simulink model "bldc_sim_2024a_v3"  (R2024a)
settings: Solver=VariableStepAuto  StartTime=0.0  StopTime=0.5  FixedStep=1e-6  MaxStep=1e-4  RelTol=1e-3
values from neighbouring files (symbols this model uses):
  D_m = 1e-5    (= 1e-05)    [setup_motor_params.m]
  J = 12e-4    (= 0.0012)    [setup_motor_params.m]
  L_ss = 0.45e-3    (= 0.00045)    [setup_motor_params.m]
  lambda_m = 21.5e-3    (= 0.0215)    [setup_motor_params.m]
  P = 8    [setup_motor_params.m]
  phi_A_deg = 9.0 * 0    (= 0)    [setup_motor_params.m]
  phi_B_deg = -1.0 * 0    (= 0)    [setup_motor_params.m]
  phi_C_deg = 7.0* 0    (= 0)    [setup_motor_params.m]
  R_s = 0.15    [setup_motor_params.m]
  tau_s = L_ss/R_s    (= 0.003)    [setup_motor_params.m]
  Ts_motor = 1e-6    (= 1e-06)    [setup_motor_params.m]
undefined symbols (not defined in the file or in its folder): closed_loop, R_vs, V_bus
libraries: spsMosfetLib x6, spsSeriesRLCBranchLib x4, spsPWMGeneratorDCDCLib x3, spsVoltageMeasurementLib x3, spsControlledCurrentSourceLib x3, spsDCVoltageSourceLib x1, spspowerguiLib x1
settings Model: Creator=Aether  LastModifiedBy=Aether

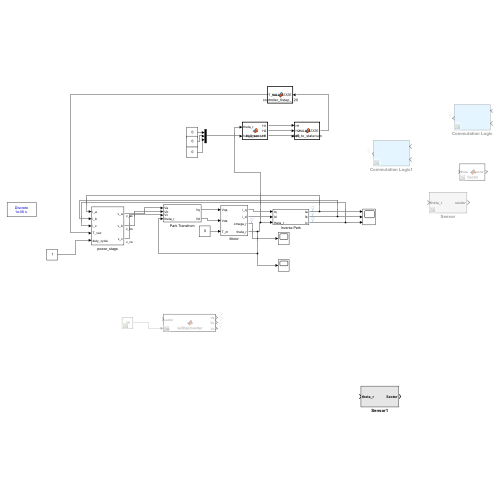
[thumbnail: Simulink's stored preview of the top-level diagram]
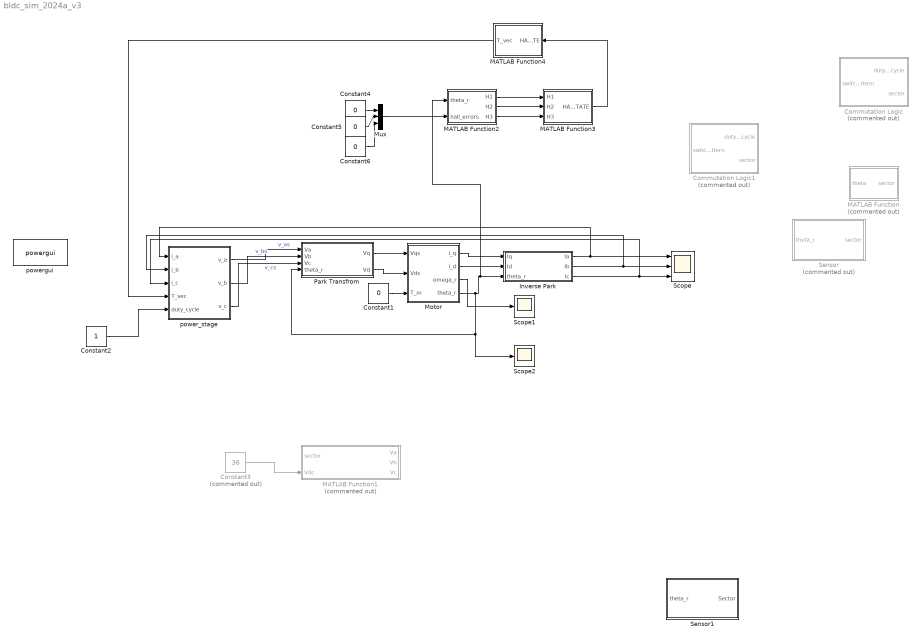
== system bldc_sim_2024a_v3 ==
  Commutation Logic : Subsystem  Commented=on
  Commutation Logic1 : Subsystem  Commented=on
  Constant{1,4..6} (4 alike) : Constant  Value=0
  Constant2 : Constant
  Constant3 : Constant  Commented=on  Value=36
  Inverse Park : Subsystem
  MATLAB Function : MATLAB Function  Commented=on  TreatAsAtomicUnit=on
  MATLAB Function1 : MATLAB Function  Commented=on  TreatAsAtomicUnit=on
  MATLAB Function2 : MATLAB Function  TreatAsAtomicUnit=on
  MATLAB Function3 : MATLAB Function  TreatAsAtomicUnit=on
  MATLAB Function4 : MATLAB Function  TreatAsAtomicUnit=on
  Motor : Subsystem
  Mux : Mux  Inputs=3
  Park Transfrom : Subsystem
  Scope : Scope  NumInputPorts=3
  Scope1 : Scope
  Scope2 : Scope
  Sensor : Subsystem  Commented=on
  Sensor1 : Subsystem
  power_stage : Subsystem
  powergui : spspowerguiLib/powergui  Priority=1  SimulationMode=Discrete  SampleTime=1e-6  frequency=60  Iterations=50  frequencyindice=0  Pbase=100e6  ErrMax=1e-4  UnitsV=kV  UnitsW=MW  buscounter=0  FunctionMessages=off  echomessages=off  EnableUseOfTLC=off  CurrentSourceSwitches=off  DisableSnubberDevices=off  DisableRonSwitches=off  DisableVfSwitches=off  DisplayEquations=off  AutomaticDiscreteSolvers=off  SolverType=Tustin/Backward Euler (TBE)  Interpol=off  ExternalGateDelay=off  methode=off  Ts=100  x0status=blocks  SPID=on  SwTol=0  HookPort=off  NonlinearTolerance=1e-4  nMaxIteration=100  ContinueOnMaxIteration=off  RestoreLinks=warning  ResistiveCurrentMeasurement=off  Frange=[0:2:500]  Ylog=off  Xlog=on  ShowGrid=off  save=off  variable=ZData  structure=0  ZoomFFT=off  StartTime=0.0  cycles=1  DisplayStyle=1  fundamental=60  FreqAxis=off  MaxFrequency=1000  frequencyindicesteady=1  RmsSteady=1  display=off
  wires:
  Park Transfrom/1(Vq) -> Motor/1(Vqs)
  Park Transfrom/2(Vd) -> Motor/2(Vds)
  Motor/1(i_q) -> Inverse Park/1(Iq)
  Motor/2(i_d) -> Inverse Park/2(Id)
  Motor/4(theta_r) -> Scope2/1, Park Transfrom/4(theta_r), MATLAB Function2/1(theta_r), Inverse Park/3(theta_r)
  Inverse Park/1(Ia) -> power_stage/1(i_a), Scope/1
  Inverse Park/2(Ib) -> power_stage/2(i_b), Scope/2
  Inverse Park/3(Ic) -> power_stage/3(i_c), Scope/3
  Constant1/1 -> Motor/3(T_m)
  Motor/3(omega_r) -> Scope1/1
  Constant3/1 -> MATLAB Function1/2(Vdc)
  MATLAB Function4/1(T_vec) -> power_stage/4(T_vec)
  Constant6/1 -> Mux/3
  Constant4/1 -> Mux/1
  MATLAB Function2/1(H1) -> MATLAB Function3/1(H1)
  Mux/1 -> MATLAB Function2/2(hall_errors)
  MATLAB Function2/3(H3) -> MATLAB Function3/3(H3)
  MATLAB Function3/1(HALL_STATE) -> MATLAB Function4/1(HALL_STATE)
  Constant5/1 -> Mux/2
  MATLAB Function2/2(H2) -> MATLAB Function3/2(H2)
  power_stage/1(v_a) -> Park Transfrom/1(Va)  "v_as"
  power_stage/2(v_b) -> Park Transfrom/2(Vb)  "v_bs"
  power_stage/3(v_c) -> Park Transfrom/3(Vc)  "v_cs"
  Constant2/1 -> power_stage/5(duty_cycle)

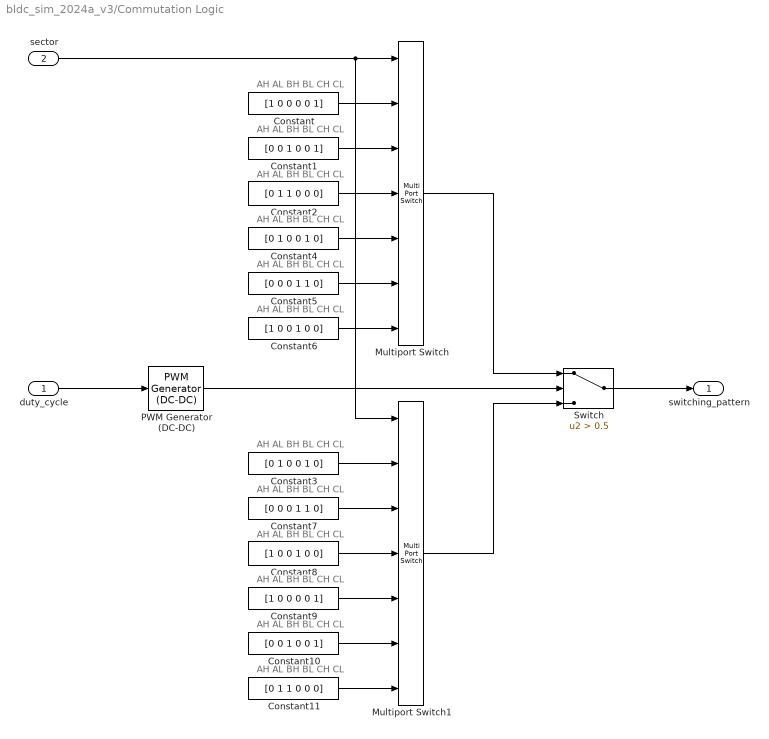
== system bldc_sim_2024a_v3/Commutation Logic ==
  note: AH AL BH BL CH CL
  note: AH AL BH BL CH CL
  note: AH AL BH BL CH CL
  note: AH AL BH BL CH CL
  note: AH AL BH BL CH CL
  note: AH AL BH BL CH CL
  note: AH AL BH BL CH CL
  note: AH AL BH BL CH CL
  note: AH AL BH BL CH CL
  note: AH AL BH BL CH CL
  note: AH AL BH BL CH CL
  note: AH AL BH BL CH CL
  duty_cycle : Inport
  sector : Inport  Port=2
  Constant : Constant  Value=[1 0 0 0 0 1]
  Constant1 : Constant  Value=[0 0 1 0 0 1]
  Constant10 : Constant  Value=[0 0 1 0 0 1]
  Constant11 : Constant  Value=[0 1 1 0 0 0]
  Constant2 : Constant  Value=[0 1 1 0 0 0]
  Constant3 : Constant  Value=[0 1 0 0 1 0]
  Constant4 : Constant  Value=[0 1 0 0 1 0]
  Constant5 : Constant  Value=[0 0 0 1 1 0]
  Constant6 : Constant  Value=[1 0 0 1 0 0]
  Constant7 : Constant  Value=[0 0 0 1 1 0]
  Constant8 : Constant  Value=[1 0 0 1 0 0]
  Constant9 : Constant  Value=[1 0 0 0 0 1]
  Multiport Switch : MultiPortSwitch  Inputs=6  SaturateOnIntegerOverflow=off  InputSameDT=off
  Multiport Switch1 : MultiPortSwitch  Inputs=6  SaturateOnIntegerOverflow=off  InputSameDT=off
  PWM Generator (DC-DC) : spsPWMGeneratorDCDCLib/PWM Generator (DC-DC)  Fsw=1e4  Ts=Ts_motor
  Switch : Switch  Criteria=u2 > Threshold  Threshold=0.5  SaturateOnIntegerOverflow=off  InputSameDT=off
  "  switching_pattern" : Outport  VectorParamsAs1DForOutWhenUnconnected=off
  wires:
  Constant6/1 -> Multiport Switch/7
  Constant4/1 -> Multiport Switch/5
  sector/1 -> Multiport Switch1/1, Multiport Switch/1
  Constant1/1 -> Multiport Switch/3
  Constant2/1 -> Multiport Switch/4
  Constant5/1 -> Multiport Switch/6
  Constant/1 -> Multiport Switch/2
  Constant9/1 -> Multiport Switch1/5
  Constant11/1 -> Multiport Switch1/7
  Constant3/1 -> Multiport Switch1/2
  Constant7/1 -> Multiport Switch1/3
  Constant10/1 -> Multiport Switch1/6
  Constant8/1 -> Multiport Switch1/4
  PWM Generator (DC-DC)/1 -> Switch/2
  Switch/1 -> "  switching_pattern"/1
  Multiport Switch/1 -> Switch/1
  Multiport Switch1/1 -> Switch/3
  duty_cycle/1 -> PWM Generator (DC-DC)/1

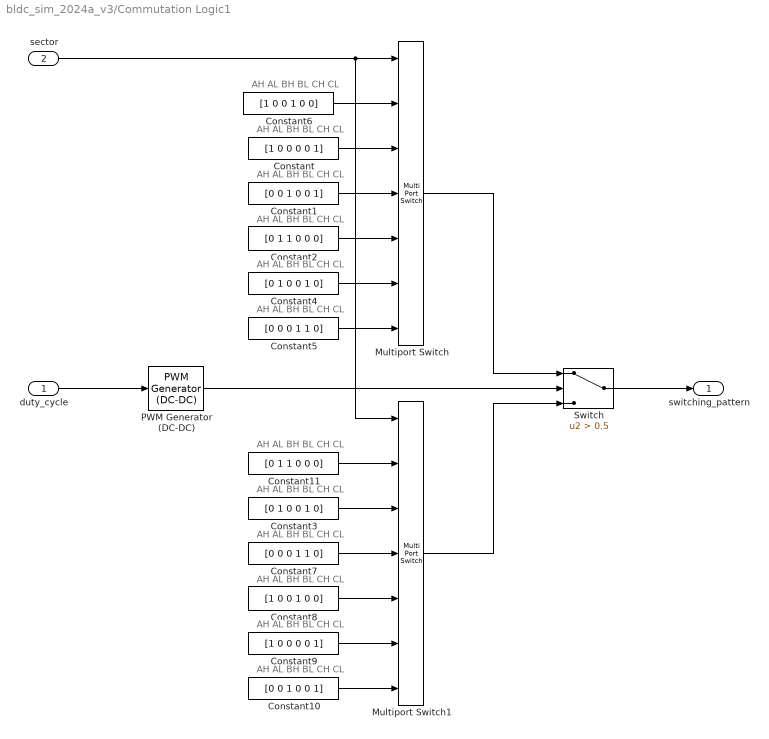
== system bldc_sim_2024a_v3/Commutation Logic1 ==
  note: AH AL BH BL CH CL
  note: AH AL BH BL CH CL
  note: AH AL BH BL CH CL
  note: AH AL BH BL CH CL
  note: AH AL BH BL CH CL
  note: AH AL BH BL CH CL
  note: AH AL BH BL CH CL
  note: AH AL BH BL CH CL
  note: AH AL BH BL CH CL
  note: AH AL BH BL CH CL
  note: AH AL BH BL CH CL
  note: AH AL BH BL CH CL
  duty_cycle : Inport
  sector : Inport  Port=2
  Constant : Constant  Value=[1 0 0 0 0 1]
  Constant1 : Constant  Value=[0 0 1 0 0 1]
  Constant10 : Constant  Value=[0 0 1 0 0 1]
  Constant11 : Constant  Value=[0 1 1 0 0 0]
  Constant2 : Constant  Value=[0 1 1 0 0 0]
  Constant3 : Constant  Value=[0 1 0 0 1 0]
  Constant4 : Constant  Value=[0 1 0 0 1 0]
  Constant5 : Constant  Value=[0 0 0 1 1 0]
  Constant6 : Constant  Value=[1 0 0 1 0 0]
  Constant7 : Constant  Value=[0 0 0 1 1 0]
  Constant8 : Constant  Value=[1 0 0 1 0 0]
  Constant9 : Constant  Value=[1 0 0 0 0 1]
  Multiport Switch : MultiPortSwitch  Inputs=6  SaturateOnIntegerOverflow=off  InputSameDT=off
  Multiport Switch1 : MultiPortSwitch  Inputs=6  SaturateOnIntegerOverflow=off  InputSameDT=off
  PWM Generator (DC-DC) : spsPWMGeneratorDCDCLib/PWM Generator (DC-DC)  Fsw=1e4  Ts=Ts_motor
  Switch : Switch  Criteria=u2 > Threshold  Threshold=0.5  SaturateOnIntegerOverflow=off  InputSameDT=off
  "  switching_pattern" : Outport  VectorParamsAs1DForOutWhenUnconnected=off
  wires:
  sector/1 -> Multiport Switch1/1, Multiport Switch/1
  PWM Generator (DC-DC)/1 -> Switch/2
  Switch/1 -> "  switching_pattern"/1
  Multiport Switch/1 -> Switch/1
  Multiport Switch1/1 -> Switch/3
  duty_cycle/1 -> PWM Generator (DC-DC)/1
  Constant5/1 -> Multiport Switch/7
  Constant4/1 -> Multiport Switch/6
  Constant2/1 -> Multiport Switch/5
  Constant1/1 -> Multiport Switch/4
  Constant/1 -> Multiport Switch/3
  Constant6/1 -> Multiport Switch/2
  Constant10/1 -> Multiport Switch1/7
  Constant9/1 -> Multiport Switch1/6
  Constant8/1 -> Multiport Switch1/5
  Constant7/1 -> Multiport Switch1/4
  Constant3/1 -> Multiport Switch1/3
  Constant11/1 -> Multiport Switch1/2

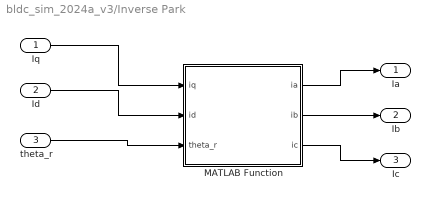
== system bldc_sim_2024a_v3/Inverse Park ==
  Iq : Inport
  Id : Inport  Port=2
  theta_r : Inport  Port=3
  MATLAB Function : MATLAB Function  TreatAsAtomicUnit=on
  Ia : Outport
  Ib : Outport  Port=2
  Ic : Outport  Port=3
  wires:
  theta_r/1 -> MATLAB Function/3(theta_r)
  Id/1 -> MATLAB Function/2(id)
  Iq/1 -> MATLAB Function/1(iq)
  MATLAB Function/3(ic) -> Ic/1
  MATLAB Function/1(ia) -> Ia/1
  MATLAB Function/2(ib) -> Ib/1

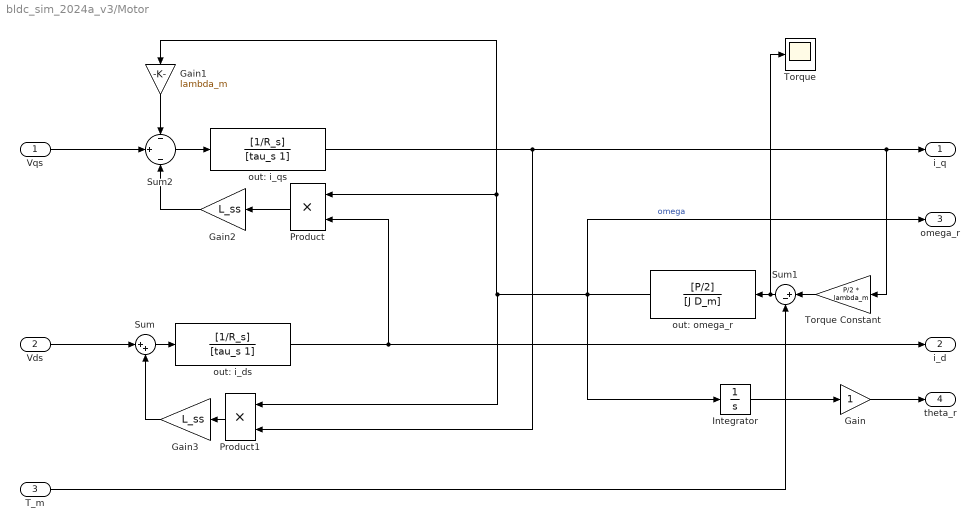
== system bldc_sim_2024a_v3/Motor ==
  Vqs : Inport
  Vds : Inport  Port=2
  T_m : Inport  Port=3
  Gain : Gain
  Gain1 : Gain  Gain=lambda_m
  Gain2 : Gain  Gain=L_ss
  Gain3 : Gain  Gain=L_ss
  Integrator : Integrator
  Product : Product
  Product1 : Product
  Sum : Sum  Inputs=|++
  Sum1 : Sum  Inputs=|+-
  Sum2 : Sum  Inputs=-|+|-
  Torque : Scope
  Torque Constant : Gain  Gain=P/2 * lambda_m
  out: i_ds : TransferFcn  Numerator=[1/R_s]  Denominator=[tau_s 1]
  out: i_qs : TransferFcn  Numerator=[1/R_s]  Denominator=[tau_s 1]
  out: omega_r : TransferFcn  Numerator=[P/2]  Denominator=[J D_m]
  i_q : Outport
  i_d : Outport  Port=2
  omega_r : Outport  Port=3
  theta_r : Outport  Port=4
  wires:
  Sum2/1 -> out: i_qs/1
  Vqs/1 -> Sum2/2
  out: omega_r/1 -> omega_r/1, Integrator/1, Product1/1, Product/1, Gain1/1  "omega"
  Gain1/1 -> Sum2/1
  out: i_ds/1 -> Product/2, i_d/1
  Integrator/1 -> Gain/1
  T_m/1 -> Sum1/2
  Sum1/1 -> Torque/1, out: omega_r/1
  Sum/1 -> out: i_ds/1
  Torque Constant/1 -> Sum1/1
  Product/1 -> Gain2/1
  out: i_qs/1 -> Product1/2, i_q/1, Torque Constant/1
  Vds/1 -> Sum/1
  Gain/1 -> theta_r/1
  Product1/1 -> Gain3/1
  Gain3/1 -> Sum/2
  Gain2/1 -> Sum2/3

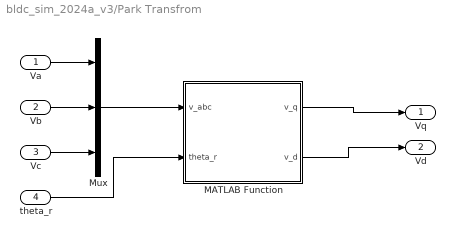
== system bldc_sim_2024a_v3/Park Transfrom ==
  Va : Inport
  Vb : Inport  Port=2
  Vc : Inport  Port=3
  theta_r : Inport  Port=4
  MATLAB Function : MATLAB Function  TreatAsAtomicUnit=on
  Mux : Mux  Inputs=3
  Vq : Outport
  Vd : Outport  Port=2
  wires:
  theta_r/1 -> MATLAB Function/2(theta_r)
  Vb/1 -> Mux/2
  Va/1 -> Mux/1
  Vc/1 -> Mux/3
  Mux/1 -> MATLAB Function/1(v_abc)
  MATLAB Function/2(v_d) -> Vd/1
  MATLAB Function/1(v_q) -> Vq/1

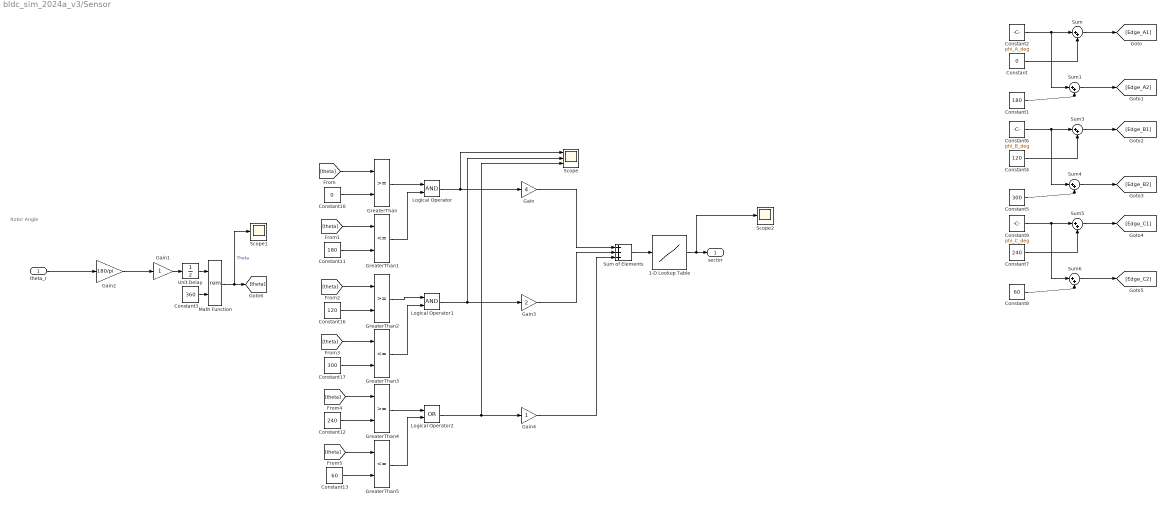
== system bldc_sim_2024a_v3/Sensor ==
  note: Rotor Angle
  theta_r : Inport
  1-D Lookup Table : Lookup_n-D  NumberOfTableDimensions=1  BreakpointsForDimension1=[1 2 3 4 5 6]  Table=[6 4 5 2 1 3]  ExtrapMethod=Clip  InternalRulePriority=Speed  RndMeth=Simplest
  Constant : Constant  Value=0
  Constant1 : Constant  Value=180
  Constant10 : Constant  Value=0
  Constant11 : Constant  Value=180
  Constant12 : Constant  Value=240
  Constant13 : Constant  Value=60
  Constant16 : Constant  Value=120
  Constant17 : Constant  Value=300
  Constant2 : Constant  Value=phi_A_deg
  Constant3 : Constant  Value=360
  Constant4 : Constant  Value=120
  Constant5 : Constant  Value=300
  Constant6 : Constant  Value=phi_B_deg
  Constant7 : Constant  Value=240
  Constant8 : Constant  Value=60
  Constant9 : Constant  Value=phi_C_deg
  Gain : Gain  Gain=4
  Gain1 : Gain
  Gain2 : Gain  Gain=180/pi
  Gain3 : Gain  Gain=2
  Gain4 : Gain
  GreaterThan : RelationalOperator  OutDataTypeStr=boolean  RndMeth=Simplest  InputSameDT=off
  GreaterThan1 : RelationalOperator  Operator=<=  OutDataTypeStr=boolean  RndMeth=Simplest  InputSameDT=off
  GreaterThan2 : RelationalOperator  OutDataTypeStr=boolean  RndMeth=Simplest  InputSameDT=off
  GreaterThan3 : RelationalOperator  Operator=<=  OutDataTypeStr=boolean  RndMeth=Simplest  InputSameDT=off
  GreaterThan4 : RelationalOperator  OutDataTypeStr=boolean  RndMeth=Simplest  InputSameDT=off
  GreaterThan5 : RelationalOperator  Operator=<=  OutDataTypeStr=boolean  RndMeth=Simplest  InputSameDT=off
  Logical Operator : Logic  AllPortsSameDT=off  OutDataTypeStr=boolean
  Logical Operator1 : Logic  AllPortsSameDT=off  OutDataTypeStr=boolean
  Logical Operator2 : Logic  Operator=OR  AllPortsSameDT=off  OutDataTypeStr=boolean
  Math Function : Math  Operator=rem  SignedPower=on
  Scope : Scope  NumInputPorts=3
  Scope1 : Scope
  Scope2 : Scope
  Sum{,1,3..6} (6 alike) : Sum  Inputs=|++
  Sum of Elements : Sum  Inputs=+++
  Unit Delay : UnitDelay  SampleTime=Ts_motor  HasFrameUpgradeWarning=on
  sector : Outport
  wires:
  Gain2/1 -> Gain1/1
  Constant3/1 -> Math Function/2
  Gain1/1 -> Unit Delay/1
  Unit Delay/1 -> Math Function/1
  Constant/1 -> Sum/2
  Constant2/1 -> Sum1/1, Sum/1
  Constant1/1 -> Sum1/2
  Sum/1 -> [Edge_A1]
  Sum1/1 -> [Edge_A2]
  Constant6/1 -> Sum4/1, Sum3/1
  Constant5/1 -> Sum4/2
  Constant4/1 -> Sum3/2
  Sum3/1 -> [Edge_B1]
  Sum4/1 -> [Edge_B2]
  Constant9/1 -> Sum6/1, Sum5/1
  Constant8/1 -> Sum6/2
  Constant7/1 -> Sum5/2
  Sum5/1 -> [Edge_C1]
  Sum6/1 -> [Edge_C2]
  theta_r/1 -> Gain2/1
  Math Function/1 -> Scope1/1, [theta]  "Theta"
  GreaterThan/1 -> Logical Operator/1
  [theta] -> GreaterThan/1
  Constant11/1 -> GreaterThan1/2
  GreaterThan1/1 -> Logical Operator/2
  GreaterThan3/1 -> Logical Operator1/2
  GreaterThan2/1 -> Logical Operator1/1
  GreaterThan4/1 -> Logical Operator2/1
  GreaterThan5/1 -> Logical Operator2/2
  Logical Operator/1 -> Scope/1, Gain/1
  Logical Operator1/1 -> Scope/2, Gain3/1
  Logical Operator2/1 -> Scope/3, Gain4/1
  Sum of Elements/1 -> 1-D Lookup Table/1
  Gain/1 -> Sum of Elements/1
  Gain3/1 -> Sum of Elements/2
  Gain4/1 -> Sum of Elements/3
  1-D Lookup Table/1 -> Scope2/1, sector/1
  Constant10/1 -> GreaterThan/2
  [theta] -> GreaterThan1/1
  [theta] -> GreaterThan2/1
  Constant16/1 -> GreaterThan2/2
  [theta] -> GreaterThan3/1
  Constant17/1 -> GreaterThan3/2
  [theta] -> GreaterThan4/1
  Constant12/1 -> GreaterThan4/2
  [theta] -> GreaterThan5/1
  Constant13/1 -> GreaterThan5/2

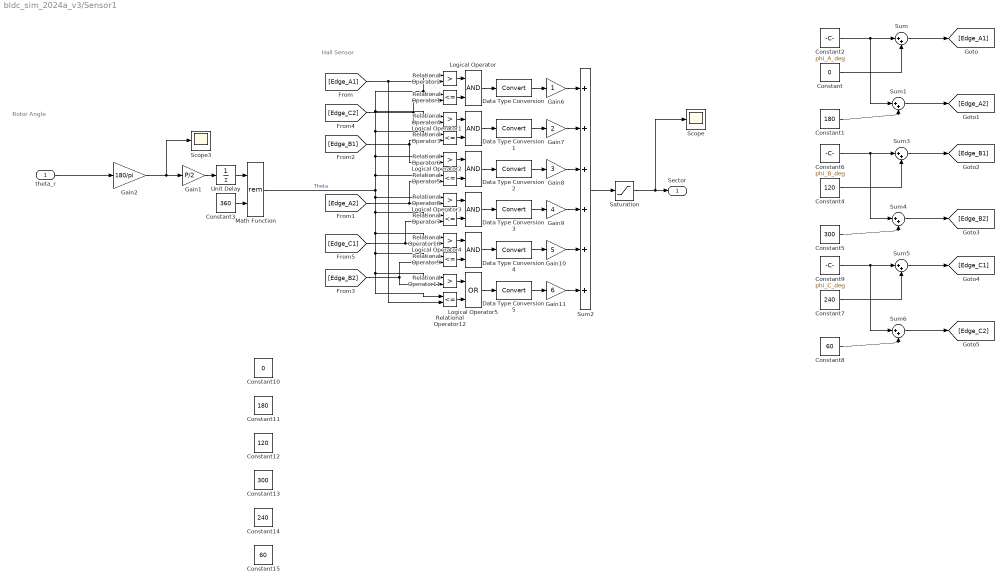
== system bldc_sim_2024a_v3/Sensor1 ==
  note: Rotor Angle
  note: Hall Sensor
  theta_r : Inport
  Constant : Constant  Value=0
  Constant1 : Constant  Value=180
  Constant10 : Constant  Value=0
  Constant11 : Constant  Value=180
  Constant12 : Constant  Value=120
  Constant13 : Constant  Value=300
  Constant14 : Constant  Value=240
  Constant15 : Constant  Value=60
  Constant2 : Constant  Value=phi_A_deg
  Constant3 : Constant  Value=360
  Constant4 : Constant  Value=120
  Constant5 : Constant  Value=300
  Constant6 : Constant  Value=phi_B_deg
  Constant7 : Constant  Value=240
  Constant8 : Constant  Value=60
  Constant9 : Constant  Value=phi_C_deg
  Data Type Conversion{,1..5} (6 alike) : DataTypeConversion
  Gain1 : Gain  Gain=P/2
  Gain10 : Gain  Gain=5  SaturateOnIntegerOverflow=on  OutDataTypeStr=Inherit: Same as input  ParamDataTypeStr=Inherit: Same as input
  Gain11 : Gain  Gain=6  SaturateOnIntegerOverflow=on  OutDataTypeStr=Inherit: Same as input  ParamDataTypeStr=Inherit: Same as input
  Gain2 : Gain  Gain=180/pi
  Gain6 : Gain  SaturateOnIntegerOverflow=on  OutDataTypeStr=Inherit: Same as input  ParamDataTypeStr=Inherit: Same as input
  Gain7 : Gain  Gain=2  SaturateOnIntegerOverflow=on  OutDataTypeStr=Inherit: Same as input  ParamDataTypeStr=Inherit: Same as input
  Gain8 : Gain  Gain=3  SaturateOnIntegerOverflow=on  OutDataTypeStr=Inherit: Same as input  ParamDataTypeStr=Inherit: Same as input
  Gain9 : Gain  Gain=4  SaturateOnIntegerOverflow=on  OutDataTypeStr=Inherit: Same as input  ParamDataTypeStr=Inherit: Same as input
  Logical Operator{,1..4} (5 alike) : Logic
  Logical Operator5 : Logic  Operator=OR
  Math Function : Math  Operator=rem  SignedPower=on
  Relational Operator{1,3,5,7,9,12} (6 alike) : RelationalOperator  Operator=<=
  Relational Operator{2,4,6,8,10..11} (6 alike) : RelationalOperator  Operator=>
  Saturation : Saturate  UpperLimit=6  LowerLimit=1
  Scope : Scope
  Scope3 : Scope
  Sum{,1,3..6} (6 alike) : Sum  Inputs=|++
  Sum2 : Sum  Inputs=++++++  InputSameDT=on  SaturateOnIntegerOverflow=on  OutDataTypeStr=Inherit: Same as first input
  Unit Delay : UnitDelay  SampleTime=Ts_motor  HasFrameUpgradeWarning=on
  Sector : Outport
  wires:
  Saturation/1 -> Scope/1, Sector/1
  Math Function/1 -> Relational Operator2/1, Relational Operator1/1, Relational Operator4/1, Relational Operator3/1, Relational Operator6/1, Relational Operator5/1, Relational Operator12/1, Relational Operator11/1, Relational Operator9/1, Relational Operator10/1, Relational Operator7/1, Relational Operator8/1  "Theta"
  Data Type Conversion5/1 -> Gain11/1
  Data Type Conversion4/1 -> Gain10/1
  Data Type Conversion3/1 -> Gain9/1
  Data Type Conversion2/1 -> Gain8/1
  Data Type Conversion1/1 -> Gain7/1
  Data Type Conversion/1 -> Gain6/1
  Relational Operator2/1 -> Logical Operator/1
  Relational Operator1/1 -> Logical Operator/2
  Logical Operator/1 -> Data Type Conversion/1
  [Edge_A1] -> Relational Operator12/2, Relational Operator2/2
  Relational Operator4/1 -> Logical Operator1/1
  Relational Operator3/1 -> Logical Operator1/2
  Logical Operator1/1 -> Data Type Conversion1/1
  [Edge_C2] -> Relational Operator1/2, Relational Operator4/2
  Relational Operator6/1 -> Logical Operator2/1
  Relational Operator5/1 -> Logical Operator2/2
  Logical Operator2/1 -> Data Type Conversion2/1
  Relational Operator8/1 -> Logical Operator3/1
  Relational Operator7/1 -> Logical Operator3/2
  Logical Operator3/1 -> Data Type Conversion3/1
  Relational Operator10/1 -> Logical Operator4/1
  Relational Operator9/1 -> Logical Operator4/2
  Logical Operator4/1 -> Data Type Conversion4/1
  Relational Operator11/1 -> Logical Operator5/1
  Relational Operator12/1 -> Logical Operator5/2
  Logical Operator5/1 -> Data Type Conversion5/1
  Gain6/1 -> Sum2/1
  Gain7/1 -> Sum2/2
  Gain8/1 -> Sum2/3
  Gain9/1 -> Sum2/4
  Gain10/1 -> Sum2/5
  Gain11/1 -> Sum2/6
  Sum2/1 -> Saturation/1
  Gain2/1 -> Scope3/1, Gain1/1
  Constant3/1 -> Math Function/2
  Gain1/1 -> Unit Delay/1
  Unit Delay/1 -> Math Function/1
  Constant/1 -> Sum/2
  Constant2/1 -> Sum1/1, Sum/1
  Constant1/1 -> Sum1/2
  Sum/1 -> [Edge_A1]
  Sum1/1 -> [Edge_A2]
  Constant6/1 -> Sum4/1, Sum3/1
  Constant5/1 -> Sum4/2
  Constant4/1 -> Sum3/2
  Sum3/1 -> [Edge_B1]
  Sum4/1 -> [Edge_B2]
  Constant9/1 -> Sum6/1, Sum5/1
  Constant8/1 -> Sum6/2
  Constant7/1 -> Sum5/2
  Sum5/1 -> [Edge_C1]
  Sum6/1 -> [Edge_C2]
  [Edge_B1] -> Relational Operator3/2, Relational Operator6/2
  [Edge_A2] -> Relational Operator5/2, Relational Operator8/2
  [Edge_C1] -> Relational Operator7/2, Relational Operator10/2
  [Edge_B2] -> Relational Operator11/2, Relational Operator9/2
  theta_r/1 -> Gain2/1

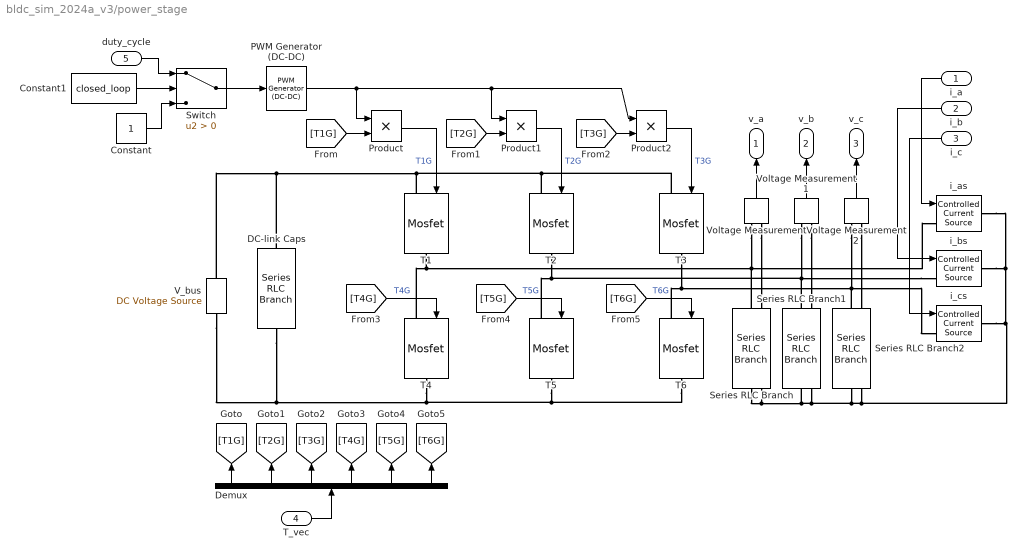
== system bldc_sim_2024a_v3/power_stage ==
  i_a : Inport
  i_b : Inport  Port=2
  i_c : Inport  Port=3
  T_vec : Inport  Port=4
  duty_cycle : Inport  Port=5
  Constant : Constant
  Constant1 : Constant  Value=closed_loop
  DC-link Caps : spsSeriesRLCBranchLib/Series RLC Branch  LConnTagsString=__new0  RConnTagsString=__new0  BranchType=RC  Resistance=1e-6  Inductance=0  SetiL0=off  InitialCurrent=0  Capacitance=100e-6  Setx0=off  InitialVoltage=0  Measurements=None
  Demux : Demux  Outputs=6
  PWM Generator (DC-DC) : spsPWMGeneratorDCDCLib/PWM Generator (DC-DC)  Fsw=f_SW_Hz  Ts=0
  Product : Product
  Product1 : Product
  Product2 : Product
  Series RLC Branch : spsSeriesRLCBranchLib/Series RLC Branch  LConnTagsString=__new0  RConnTagsString=__new0  BranchType=R  Resistance=R_vs  Inductance=0  SetiL0=off  InitialCurrent=0  Capacitance=inf  Setx0=off  InitialVoltage=0  Measurements=None
  Series RLC Branch1 : spsSeriesRLCBranchLib/Series RLC Branch  LConnTagsString=__new0  RConnTagsString=__new0  BranchType=R  Resistance=R_vs  Inductance=0  SetiL0=off  InitialCurrent=0  Capacitance=inf  Setx0=off  InitialVoltage=0  Measurements=None
  Series RLC Branch2 : spsSeriesRLCBranchLib/Series RLC Branch  LConnTagsString=__new0  RConnTagsString=__new0  BranchType=R  Resistance=R_vs  Inductance=0  SetiL0=off  InitialCurrent=0  Capacitance=inf  Setx0=off  InitialVoltage=0  Measurements=None
  Switch : Switch  Criteria=u2 > Threshold  SaturateOnIntegerOverflow=off  InputSameDT=off
  T{1..6} (6 alike) : spsMosfetLib/Mosfet  Ron=R_dsON_Ohm  Lon=0  Rd=0.01  Vfd=0.7  IC=0  Rs=1e5  Cs=inf  Measurements=off
  V_bus : spsDCVoltageSourceLib/DC Voltage Source  Amplitude=V_bus  Measurements=None
  Voltage Measurement : spsVoltageMeasurementLib/Voltage Measurement  PhasorSimulation=off  OutputType=Complex  PSBequivalent=0
  Voltage Measurement1 : spsVoltageMeasurementLib/Voltage Measurement  PhasorSimulation=off  OutputType=Complex  PSBequivalent=0
  Voltage Measurement2 : spsVoltageMeasurementLib/Voltage Measurement  PhasorSimulation=off  OutputType=Complex  PSBequivalent=0
  i_as : spsControlledCurrentSourceLib/Controlled Current Source  Initialize=on  Source_Type=AC  Amplitude=0  Phase=0  Frequency=0  Measurements=None
  i_bs : spsControlledCurrentSourceLib/Controlled Current Source  Initialize=on  Source_Type=AC  Amplitude=0  Phase=0  Frequency=0  Measurements=None
  i_cs : spsControlledCurrentSourceLib/Controlled Current Source  Initialize=on  Source_Type=AC  Amplitude=0  Phase=0  Frequency=0  Measurements=None
  v_a : Outport
  v_b : Outport  Port=2
  v_c : Outport  Port=3
  wires:
  T_vec/1 -> Demux/1
  Product1/1 -> T2/1  "T2G"
  PWM Generator (DC-DC)/1 -> Product/1, Product2/1, Product1/1
  Demux/6 -> [T6G]
  [T4G] -> T4/1  "T4G"
  [T5G] -> T5/1  "T5G"
  Demux/4 -> [T4G]
  Voltage Measurement/1 -> v_a/1
  [T2G] -> Product1/2
  Voltage Measurement1/1 -> v_b/1
  Voltage Measurement2/1 -> v_c/1
  i_a/1 -> i_as/1
  Demux/1 -> [T1G]
  Demux/5 -> [T5G]
  [T6G] -> T6/1  "T6G"
  i_c/1 -> i_cs/1
  Product/1 -> T1/1  "T1G"
  [T3G] -> Product2/2
  i_b/1 -> i_bs/1
  Product2/1 -> T3/1  "T3G"
  Demux/2 -> [T2G]
  Demux/3 -> [T3G]
  [T1G] -> Product/2
  duty_cycle/1 -> Switch/1
  Constant/1 -> Switch/3
  Constant1/1 -> Switch/2
  Switch/1 -> PWM Generator (DC-DC)/1
  connections:
  i_bs/LConn1 -- Voltage Measurement1/LConn1 -- Series RLC Branch1/LConn1 -- T2/RConn1 -- T5/LConn1
  DC-link Caps/RConn1 -- V_bus/LConn1 -- T4/RConn1 -- T6/RConn1 -- T5/RConn1
  DC-link Caps/LConn1 -- V_bus/RConn1 -- T1/LConn1 -- T3/LConn1 -- T2/LConn1
  T4/LConn1 -- T1/RConn1 -- Voltage Measurement/LConn1 -- Series RLC Branch/LConn1 -- i_as/LConn1
  T3/RConn1 -- T6/LConn1 -- Voltage Measurement2/LConn1 -- Series RLC Branch2/LConn1 -- i_cs/LConn1
  Series RLC Branch/RConn1 -- Voltage Measurement/LConn2 -- i_bs/RConn1 -- i_as/RConn1 -- i_cs/RConn1 -- Voltage Measurement2/LConn2 -- Series RLC Branch2/RConn1 -- Voltage Measurement1/LConn2 -- Series RLC Branch1/RConn1

== matlab function bldc_sim_2024a_v3/Inverse Park/MATLAB Function ==
  data: iq input; id input; ia output; theta_r input; ib output; ic output
function [ia, ib, ic] = inverse_park_transform(iq, id,theta_r)


th = theta_r;

K_inv = [ cos(th)                  sin(th);
          cos(th - 2*pi/3)         sin(th - 2*pi/3);
          cos(th + 2*pi/3)         sin(th + 2*pi/3) ];

i_dq = [iq; id];
i_abc = K_inv * i_dq;
ia = i_abc(1);
ib = i_abc(2);
ic = i_abc(3);

% a = 2*pi/3;
% K_inv = [cos(theta), sin(theta);
%          cos(theta-a), sin(theta-a);
%          cos(theta+a), sin(theta+a)];
% fqd_vec = [fq; fd];
% fs_vec = K_inv*fqd_vec;
% fa = fs_vec(1);
% fb = fs_vec(2);
% fc = fs_vec(3);


end

== matlab function bldc_sim_2024a_v3/Park Transfrom/MATLAB Function ==
  data: v_abc input; v_q output; theta_r input; v_d output
function [v_q, v_d] = park_transform(v_abc,theta_r)

th = theta_r;

K = (2/3) * [ cos(th)     cos(th - 2*pi/3)     cos(th + 2*pi/3); 
              sin(th)    sin(th - 2*pi/3)    sin(th + 2*pi/3) ];

v_dq = K * v_abc;

v_q = v_dq(1);
v_d = v_dq(2);
% %   Detailed explanation goes here
% a = 2*pi/3;
% K = (2/3)*[cos(theta), cos(theta-a), cos(theta+a);
%            sin(theta), sin(theta-a), sin(theta+a)];
% fs_vec = [fa, fb, fc]';
% fqd_vec = K*fs_vec;
% fq = fqd_vec(1);
% fd = fqd_vec(2);

end

== matlab function bldc_sim_2024a_v3/MATLAB Function ==
  data: theta input; sector output
function sector = Sector(theta)

P = 8;
theta = mod(theta * P/2, 2*pi); % wrap around

if theta >= 0 && theta < pi/3
    sector = 1;
elseif theta >= pi/3 && theta < 2*pi/3
    sector = 2;
elseif theta >= 2*pi/3 && theta < pi
    sector = 3;
elseif theta >= pi && theta < 4*pi/3
    sector = 4;
elseif theta >= 4*pi/3 && theta < 5*pi/3
    sector = 5;
else
    sector = 6;
end

== matlab function bldc_sim_2024a_v3/MATLAB Function1 ==
  data: sector input; Va output; Vdc input; Vb output; Vc output
function [Va, Vb, Vc] = sixStepInverter(sector, Vdc)

    states = int8([ 1 -1  0;   % sector 1
                    1  0 -1;   % sector 2
                    0  1 -1;   % sector 3
                   -1  1  0;   % sector 4
                   -1  0  1;   % sector 5
                    0 -1  1]); % sector 6


    

    Va = double(states(sector,1)) * (Vdc/2);
    Vb = double(states(sector,2)) * (Vdc/2);
    Vc = double(states(sector,3)) * (Vdc/2);
end

== matlab function bldc_sim_2024a_v3/MATLAB Function2 ==
  data: theta_r input; H1 output; hall_errors input; H2 output; H3 output
function [H1,H2,H3] = hall_sensor(theta_r, hall_errors)
%HALL_SENSOR Obtain hall signals from electrical angle
%   Detailed explanation goes here
H1 = 0;
H2 = 0;
H3 = 0;
theta_r1 = mod(theta_r - hall_errors(1), 2*pi);
theta_r2 = mod(theta_r - hall_errors(2), 2*pi);
theta_r3 = mod(theta_r - hall_errors(3), 2*pi);

if ((0 <= theta_r1 && theta_r1 <= pi/2) || (3*pi/2 <= theta_r1 &&  theta_r1 <=2*pi))
    H1 = 1;
end
if (pi/6 <= theta_r2 && theta_r2 <=7*pi/6)
    H2 = 1;
end
if (5*pi/6 <= theta_r3 && theta_r3 <=11*pi/6)
    H3 = 1;
end
end

== matlab function bldc_sim_2024a_v3/MATLAB Function3 ==
  data: H1 input; HALL_STATE output; H2 input; H3 input
function HALL_STATE = hall_to_statenum(H1,H2,H3)
HALL_STATE = 4*H1 + 2*H2 + H3;

== matlab function bldc_sim_2024a_v3/MATLAB Function4 ==
  data: HALL_STATE input; T_vec output
function T_vec = controller_6step_120(HALL_STATE)
%CONTROLLER_6STEP_180 Summary of this function goes here
%   Detailed explanation goes here

T_vec = zeros(6,1);
% HALL_STATE = 4*H1 + 2*H2 + H3;
if (HALL_STATE > 6)
    fprintf("Hall = %.3f", HALL_STATE)
    error("Invalid hall state!!")
end

switch HALL_STATE
    case 4 % State I
        T_vec([1,5]) = 1;
    case 6 % State II
        T_vec([1,6]) = 1;
    case 2 % State III
        T_vec([2,6]) = 1;
    case 3 % State IV
        T_vec([2,4]) = 1;
    case 1 % State V
        T_vec([3,4]) = 1;
    case 5 % State VI
        T_vec([3,5]) = 1;
    otherwise
end
end
